simulink library "RobotX_Lib"  (R2023b)
settings: Solver=VariableStepAuto  StartTime=0.0  StopTime=10.0  RelTol=1e-3
settings Model: Creator=margaridaestrela  LastModifiedBy=margaridaestrela

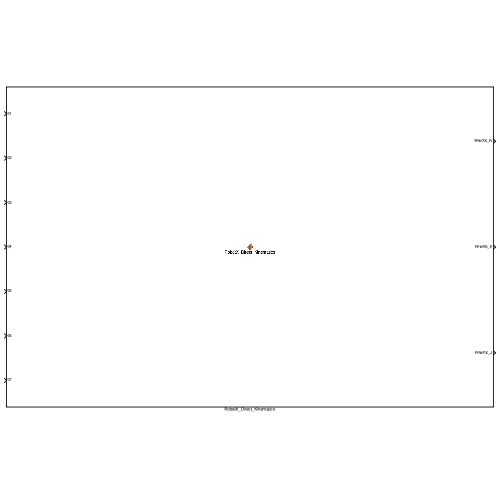
[thumbnail: Simulink's stored preview of the top-level diagram]
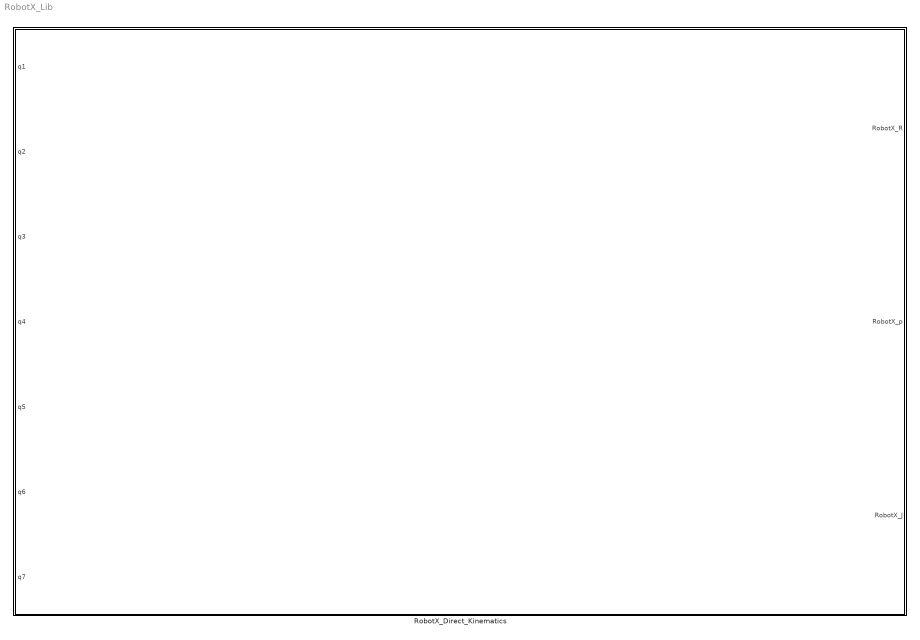
== system RobotX_Lib ==
  RobotX_Direct_Kinematics : MATLAB Function  TreatAsAtomicUnit=on

== matlab function RobotX_Lib/RobotX_Direct_Kinematics ==
  data: q1 input; q2 input; q3 input; q4 input; q5 input; RobotX_R output; q6 input; RobotX_p output; RobotX_J output; q7 input
function [RobotX_R,RobotX_p,RobotX_J] = RobotX_Direct_Kinematics(q1,q2,q3,q4,q5,q6,q7)
%#codegen

%    This function was generated by the Symbolic Math Toolbox version 23.2.
%    07-May-2024 11:22:48

% q1 = complex(q1);  % if required to enforce complex operations
% q2 = complex(q2);  % if required to enforce complex operations
% q3 = complex(q3);  % if required to enforce complex operations
% q4 = complex(q4);  % if required to enforce complex operations
% q5 = complex(q5);  % if required to enforce complex operations
% q6 = complex(q6);  % if required to enforce complex operations
% q7 = complex(q7);  % if required to enforce complex operations
t2 = cos(q2);
t3 = cos(q3);
t4 = cos(q4);
t5 = cos(q5);
t6 = cos(q6);
t7 = cos(q7);
t8 = sin(q2);
t9 = sin(q3);
t10 = sin(q4);
t11 = sin(q5);
t12 = sin(q6);
t13 = sin(q7);
t14 = q3+q4;
t18 = -q1;
t15 = t2.*5.0;
t16 = cos(t14);
t17 = sin(t14);
t19 = t2.*t5;
t20 = t5.*t8;
t21 = t2.*2.5e+1;
t22 = t8.*2.5e+1;
t23 = t3.*3.15e+2;
t24 = t3.*t4.*3.5e+1;
t26 = t2.*t9.*6.3e+1;
t27 = t9.*t10.*3.5e+1;
t29 = t2.*t6.*t11;
t31 = t6.*t8.*t11;
t33 = t2.*t9.*3.15e+2;
t34 = t3.*t10.*3.65e+2;
t35 = t4.*t9.*3.65e+2;
t36 = t8.*t9.*3.15e+2;
t37 = t2.*t3.*t10.*7.0;
t38 = t2.*t4.*t9.*7.0;
t39 = t8.*t11.*t12.*1.6e+1;
t43 = t2.*t3.*t10.*t11;
t44 = t2.*t4.*t9.*t11;
t45 = t3.*t8.*t10.*t11;
t46 = t4.*t8.*t9.*t11;
t48 = t2.*t3.*t10.*3.5e+1;
t49 = t2.*t4.*t9.*3.5e+1;
t50 = t3.*t8.*t10.*3.5e+1;
t51 = t4.*t8.*t9.*3.5e+1;
t53 = t8.*t11.*t12.*8.0e+1;
t54 = t8.*t9.*t10.*3.65e+2;
t55 = t2.*t3.*t4.*7.3e+1;
t56 = t2.*t3.*t4.*3.65e+2;
t57 = t3.*t6.*t10.*8.0e+1;
t58 = t4.*t6.*t9.*8.0e+1;
t59 = t3.*t4.*t8.*3.65e+2;
t60 = t2.*t9.*t10.*7.3e+1;
t61 = t2.*t11.*t12.*8.0e+1;
t62 = t2.*t9.*t10.*3.65e+2;
t70 = t2.*t3.*t4.*t6.*1.6e+1;
t71 = t2.*t6.*t9.*t10.*1.6e+1;
t74 = t2.*t3.*t4.*t6.*8.0e+1;
t75 = t3.*t4.*t6.*t8.*8.0e+1;
t76 = t3.*t4.*t5.*t12.*8.0e+1;
t78 = t2.*t6.*t9.*t10.*8.0e+1;
t79 = t6.*t8.*t9.*t10.*8.0e+1;
t80 = t5.*t9.*t10.*t12.*8.0e+1;
t25 = -t20;
t28 = -t23;
t30 = t12.*t17;
t32 = -t24;
t40 = t5.*t6.*t16;
t41 = t2.*t12.*t16;
t42 = t8.*t12.*t16;
t47 = -t29;
t52 = -t39;
t63 = -t53;
t64 = -t54;
t65 = t3.*t6.*t10.*t19;
t66 = t4.*t6.*t9.*t19;
t67 = t3.*t6.*t10.*t20;
t68 = t4.*t6.*t9.*t20;
t72 = -t60;
t73 = -t62;
t77 = -t71;
t81 = t3.*t10.*t12.*t19.*1.6e+1;
t82 = t4.*t9.*t12.*t19.*1.6e+1;
t83 = -t78;
t84 = -t79;
t85 = -t80;
t88 = t3.*t10.*t12.*t19.*8.0e+1;
t89 = t4.*t9.*t12.*t19.*8.0e+1;
t90 = t3.*t10.*t12.*t20.*8.0e+1;
t91 = t4.*t9.*t12.*t20.*8.0e+1;
t97 = t19+t45+t46;
t69 = -t40;
t86 = -t81;
t87 = -t82;
t92 = -t88;
t93 = -t89;
t94 = -t90;
t95 = -t91;
t98 = t25+t43+t44;
t99 = t31+t41+t65+t66;
t100 = t42+t47+t67+t68;
t101 = t27+t28+t32+t34+t35+t57+t58+t76+t85+7.56e+2;
t96 = t30+t69;
RobotX_R = reshape([t7.*t100-t13.*t97,-t7.*t99+t13.*t98,t7.*t96+t11.*t13.*t16,-t7.*t97-t13.*t100,t7.*t98+t13.*t99,-t13.*t96+t7.*t11.*t16,t12.*(-t2.*t11+t3.*t10.*t20+t4.*t9.*t20)-t6.*t8.*t16,-t12.*(t8.*t11+t3.*t10.*t19+t4.*t9.*t19)+t2.*t6.*t16,-t6.*t17-t5.*t12.*t16],[3,3]);
if nargout > 1
    t102 = t101+3.65e+2;
    t103 = t15+t26+t37+t38+t52+t55+t70+t72+t77+t86+t87;
    t104 = t18+t22+t36+t50+t51+t59+t61+t64+t75+t84+t94+t95;
    RobotX_p = [t104;-t21-t33-t48-t49+t53-t56+t62-t74+t78+t88+t89;t101];
end
if nargout > 2
    RobotX_J = reshape([0.0,0.0,1.0,0.0,0.0,0.0,t21+t33+t48+t49+t56+t63+t73+t74+t83+t92+t93,t104,0.0,0.0,0.0,1.0,-t2.*t101,-t8.*t101,t2.*t18+t11.*t12.*8.0e+1-2.5e+1,t8,-t2,0.0,t21+t28+t33+t48+t49+t56+t63+t73+t74+t83+t92+t93,t9.*-3.15e+2+t104,0.0,0.0,0.0,1.0,-t4.*t101,-t10.*t101,t10.*(t10.*7.0+t103).*-5.0-t4.*(t4.*3.5e+1-t104),t10,-t4,0.0,t5.*t102,t11.*t102,-t5.*t104+t11.*t103.*5.0,-t11,t5,0.0,-t6.*t101,-t12.*t101,t6.*t104-t12.*t103.*5.0,t12,-t6,0.0],[6,7]);
end
end
